simulink model "System_model_discrete"  (R2022a)
settings: Solver=FixedStepDiscrete  StartTime=0.0  StopTime=T_final  FixedStep=T_sample  RelTol=1e-3
values from neighbouring files (symbols this model uses):
  A1 = inv(S1)*IO*U_i.'    [run_model.m]    (also in run_model_for_perform_vs_num_attack.m)
  A2 = OI*U_i.'    [run_model.m]    (also in run_model_for_perform_vs_num_attack.m)
  A_bar_d = [0.99058344787 -0.000125476588979 -1.03572369058e-05 -0.000112840130565 -4.9197018367e-06 -1.67662830632 -0.0228026014464 -0.00188074381714 -0.019999276241 -0.0008715203213 -0.00015214348792 0.987594206485 ... (100 elements, 10x10)]    [A_bar_d.mat]
  b1p = inv(S1)*IO*U_history.'    [run_model.m]    (also in run_model_for_perform_vs_num_attack.m)
  b2p = OI*U_history.'    [run_model.m]    (also in run_model_for_perform_vs_num_attack.m)
  B_bar_d = [0.00129291786986 -6.71376007658e-08 -5.54322132914e-09 -6.10354899312e-08 -2.66151497743e-09 0.269747891814 -1.80552874589e-05 -1.49023321753e-06 -1.61887101691e-05 -7.05777435188e-07 -6.71376007665e-08 0.00108984615129 ... (190 elements, 10x19)]    [B_bar_d.mat]
  BDD_thresh = 0.05*0.6352    (= 0.03176)    [plot_perform_vs_num_attacks.m]    (also in run_model.m)
  C_obsv_d = [0 0 0 0 0 -18.3910466782 17.2834976586 0.26596429707 7.1412513587 0.0956721531682 0.757058744511 -7.14197878204 ... (190 elements, 19x10)]    [C_obsv_d.mat]
  D_obsv_d = [0 0 0 0 0 0 0 0 0 0 0 0 ... (361 elements, 19x19)]    [D_obsv_d.mat]
  e_ini_matrix = reshape(e_ini,n_meas,T1)    [run_model.m]    (also in run_model_for_perform_vs_num_attack.m)
  I = Ic +mc*d^2+2*mw*L^2+2*Im    (= 0.26903125)    [Run_this_file_for_DDWMR_model.m]    (also in run_model.m = [1;2;9;11;12;16;17]; run_model_for_perform_vs_num_attack.m = sort(randperm(n_meas,n_attack)).'; test_different_horizon_size.m = sort(randperm(n_meas,n_attack)).')
  I_attack_ini = repmat(I,1,T1)    [run_model.m]    (also in run_model_for_perform_vs_num_attack.m)
  l = n_meas    (= 19)    [run_model.m]
  load_buses = [zeros(n_gen,1); ones(n_bus-n_gen,1)]    [run_model.m]
  max_iter = 1000    [MHFDIA_Basics.m]    (also in Perform_vs_iter.m = Max_iter(idx); run_model.m = 2000; run_model_for_perform_vs_num_attack.m = 300)
  n = 5    [MHFDIA_Basics.m]    (also in discretize_linear_model.m = size(A,1); run_model.m = 10)
  n_bus = 14    [run_model.m]
  n_gen = 5    [run_model.m]
  n_meas = n_gen + n_bus    (= 19)    [run_model.m]    (also in test_different_horizon_size.m)
  Se1 = S(1:n_states,1:n_states)    [run_model.m]    (also in run_model_for_perform_vs_num_attack.m)
  T = floor(n_x/m)    [MHFDIA_Basics.m]    (also in plot_for_different_horizon_size.m = 20; run_model.m = round(2*n))
  T1 = 20    [plot_perform_vs_num_attacks.m]    (also in run_model.m; test_different_horizon_size.m = T1_array(iter))
  T_start_attack = .2*T_final    [plot_results.m]    (also in run_model.m = 1.6)
  U0 = zeros(m,T)    [run_model.m]
  Ue11 = U(I_attack(1:(T1-1)*n_attack),1:n)    [run_model.m]    (also in run_model_for_perform_vs_num_attack.m)
  Ue12 = U(I_attack((T1-1)*n_attack+1:end),1:n)    [run_model.m]    (also in run_model_for_perform_vs_num_attack.m)
  x0 = zeros(n_states,1)    [run_model.m]
  Y0 = zeros(m,T)    [run_model.m]
undefined symbols (not defined in the file or in its folder): G_T, HT, PhiT, sigbuilder_block, T_start_opt, Theta_T
libraries: simulink x5
settings Model: Creator=oanubi  LastModifiedBy=Abelb
settings SolverCC: AlgebraicLoopSolver=TrustRegion
settings DebuggingCC: UnconnectedInputMsg=warning  UnconnectedOutputMsg=warning  UnconnectedLineMsg=warning  SFMachineParentedDataDiag=warning
settings HardwareCC: TargetBitPerPointer=64  TargetBitPerSizeT=64  TargetBitPerPtrDiffT=64  TargetLongLongMode=on  TargetIntDivRoundTo=Zero  TargetEndianess=LittleEndian  TargetWordSize=64  TargetHWDeviceType=MATLAB Host  ProdEqTarget=off
settings RTWCC: Description=Create Visual C/C++ Solution File for Simulink Coder  TemplateMakefile=RTW.MSVCBuild  DLArmComputeVersion=19.05

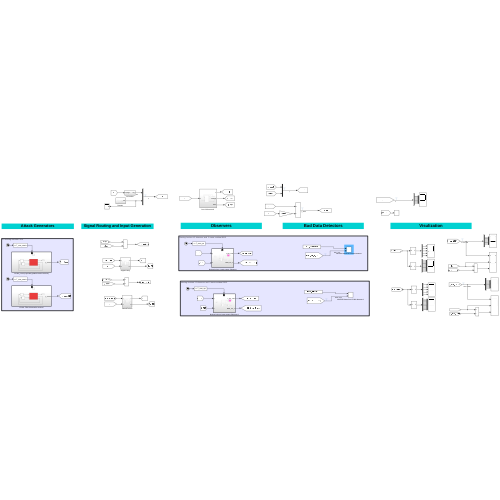
[thumbnail: Simulink's stored preview of the top-level diagram]
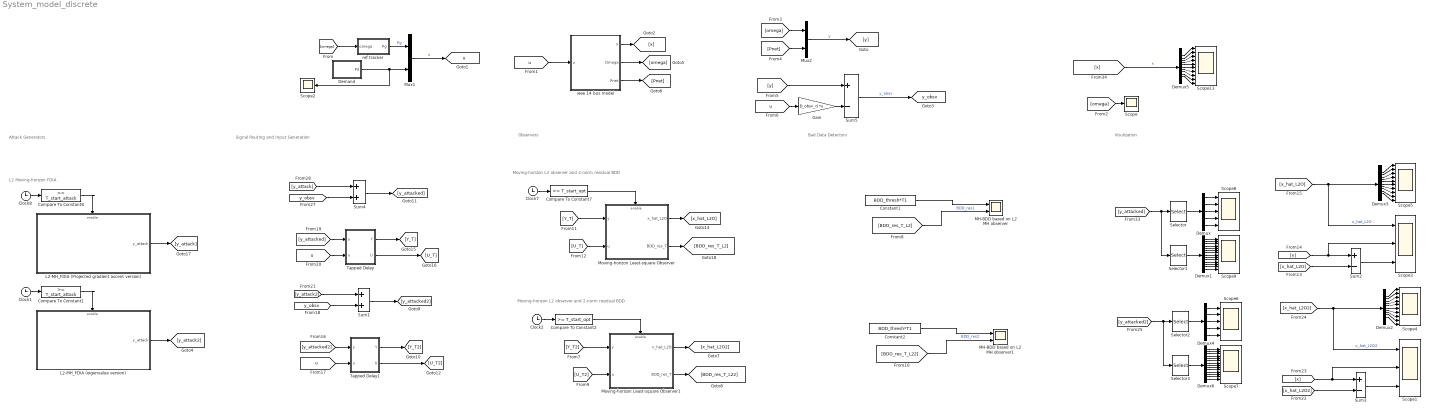
== system System_model_discrete ==
  note: L2 Moving-horizon FDIA
  note: Moving-horizon L2 observer and 2-norm residual BDD
  note: Observers
  note: Signal Routing and Input Generation
  note: Visulization
  note: Attack Generators
  note: Bad Data Detectors
  note: Moving-horizon L2 observer and 2-norm residual BDD
  Clock{1..2,7..8} (4 alike) : Clock
  Compare To Constant1 : simulink/Logic and Bit Operations/Compare To Constant  relop=>=  const=T_start_attack  OutDataTypeStr=boolean
  Compare To Constant2 : simulink/Logic and Bit Operations/Compare To Constant  relop=>=  const=T_start_opt  OutDataTypeStr=boolean
  Compare To Constant7 : simulink/Logic and Bit Operations/Compare To Constant  relop=>=  const=T_start_opt  OutDataTypeStr=boolean
  Compare To Constant8 : simulink/Logic and Bit Operations/Compare To Constant  relop=>=  const=T_start_attack  OutDataTypeStr=boolean
  Constant1 : Constant  Value=BDD_thresh*T1
  Constant2 : Constant  Value=BDD_thresh*T1
  Demand : Subsystem
  Demux : Demux  Outputs=n_gen
  Demux1 : Demux  Outputs=n_bus
  Demux2 : Demux  Outputs=n_states
  Demux3 : Demux  Outputs=n_states
  Demux4 : Demux  Outputs=n_gen
  Demux5 : Demux  Outputs=n_states
  Demux6 : Demux  Outputs=n_bus
  Gain : Gain  Gain=D_obsv_d  Multiplication=Matrix(K*u) (u vector)
  L2-MH_FDIA (Projected gradient ascent version) : Subsystem
  L2-MH_FDIA (eigenvalue version) : Subsystem
  MH-BDD based on L2 MH observer : Scope  NumInputPorts=2
  MH-BDD based on L2 MH observer1 : Scope  NumInputPorts=2
  Moving-horizon Least-square Observer : Subsystem
  Moving-horizon Least-square Observer1 : Subsystem
  Mux1 : Mux  Inputs=2
  Mux2 : Mux  Inputs=2
  Scope : Scope
  Scope1 : Scope  NumInputPorts=3
  Scope13 : Scope  NumInputPorts=10
  Scope2 : Scope
  Scope3 : Scope  NumInputPorts=3
  Scope4 : Scope  NumInputPorts=10
  Scope5 : Scope  NumInputPorts=10
  Scope6 : Scope  NumInputPorts=5
  Scope7 : Scope  NumInputPorts=14
  Scope8 : Scope  NumInputPorts=5
  Scope9 : Scope  NumInputPorts=14
  Selector : Selector  InputPortWidth=n_meas  IndexOptions=Index vector (dialog)  Indices=1:n_gen  OutputSizes=1
  Selector1 : Selector  InputPortWidth=n_meas  IndexOptions=Index vector (dialog)  Indices=n_gen+1:n_meas  OutputSizes=1
  Selector2 : Selector  InputPortWidth=n_meas  IndexOptions=Index vector (dialog)  Indices=1:n_gen  OutputSizes=1
  Selector3 : Selector  InputPortWidth=n_meas  IndexOptions=Index vector (dialog)  Indices=n_gen+1:n_meas  OutputSizes=1
  Sum1 : Sum
  Sum2 : Sum  Inputs=+-
  Sum3 : Sum  Inputs=+-
  Sum4 : Sum
  Sum5 : Sum  Inputs=+-
  Tapped Delay : Subsystem
  Tapped Delay1 : Subsystem
  ieee 14 bus model : Subsystem
  ref tracker : Subsystem
  tag scope: u=global, y_obsv=global
  wires:
  [u] -> ieee 14 bus model/1(u)
  Demand/1(Pd) -> Scope2/1, Mux1/2
  ref tracker/1(Pg) -> Mux1/1  "Pg"
  Mux1/1 -> [u]  "u"
  ieee 14 bus model/2(Omega) -> [omega]
  ieee 14 bus model/1(x) -> [x]
  ieee 14 bus model/3(Pnet) -> [Pnet]
  [omega] -> ref tracker/1(omega)
  [omega] -> Scope/1
  Mux2/1 -> [y]  "y"
  [omega] -> Mux2/1
  [Pnet] -> Mux2/2
  [y] -> Sum5/1
  Gain/1 -> Sum5/2
  [u] -> Gain/1
  Sum5/1 -> [y_obsv]  "y_obsv"
  [y_attacked] -> Tapped Delay/1(y)
  [u] -> Tapped Delay/2(u)
  [y_obsv] -> Sum4/2
  Sum4/1 -> [y_attacked]
  [y_attack] -> Sum4/1
  [y_attacked] -> Selector1/1, Selector/1
  Demux/1 -> Scope8/1
  Demux/2 -> Scope8/2
  Demux/3 -> Scope8/3
  Demux/4 -> Scope8/4
  Demux/5 -> Scope8/5
  Selector/1 -> Demux/1
  Selector1/1 -> Demux1/1
  Demux1/5 -> Scope9/5
  Demux1/4 -> Scope9/4
  Demux1/3 -> Scope9/3
  Demux1/2 -> Scope9/2
  Demux1/1 -> Scope9/1
  Demux1/6 -> Scope9/6
  Demux1/7 -> Scope9/7
  Demux1/8 -> Scope9/8
  Demux1/9 -> Scope9/9
  Demux1/10 -> Scope9/10
  Demux1/11 -> Scope9/11
  Demux1/12 -> Scope9/12
  Demux1/13 -> Scope9/13
  Demux1/14 -> Scope9/14
  [x] -> Demux5/1  "x"
  Demux5/10 -> Scope13/10
  Demux5/6 -> Scope13/6
  Demux5/8 -> Scope13/8
  Demux5/5 -> Scope13/5
  Demux5/3 -> Scope13/3
  Demux5/7 -> Scope13/7
  Demux5/2 -> Scope13/2
  Demux5/1 -> Scope13/1
  Demux5/4 -> Scope13/4
  Demux5/9 -> Scope13/9
  Compare To Constant7/1 -> Moving-horizon Least-square Observer/Enable
  Clock7/1 -> Compare To Constant7/1
  Moving-horizon Least-square Observer/1(x_hat_L2O) -> [x_hat_L2O]
  [x] -> Sum2/1, Scope3/2
  Demux3/3 -> Scope5/3
  Demux3/9 -> Scope5/9
  Demux3/5 -> Scope5/5
  Demux3/7 -> Scope5/7
  Demux3/6 -> Scope5/6
  Demux3/2 -> Scope5/2
  Demux3/1 -> Scope5/1
  Demux3/4 -> Scope5/4
  Demux3/10 -> Scope5/10
  Sum2/1 -> Scope3/3
  Demux3/8 -> Scope5/8
  [x_hat_L2O] -> Demux3/1, Scope3/1  "x_hat_L2O"
  [x_hat_L2O] -> Sum2/2
  Tapped Delay/1(Y) -> [Y_T]
  Tapped Delay/2(U) -> [U_T]
  [Y_T] -> Moving-horizon Least-square Observer/1(y)
  [U_T] -> Moving-horizon Least-square Observer/2(u)
  Moving-horizon Least-square Observer/2(BDD_res_T) -> [BDD_res_T_L2]
  Constant1/1 -> MH-BDD based on L2 MH observer/1
  [BDD_res_T_L2] -> MH-BDD based on L2 MH observer/2  "BDD_res1"
  L2-MH_FDIA (Projected gradient ascent version)/1(y_attack) -> [y_attack]
  Clock8/1 -> Compare To Constant8/1
  Compare To Constant8/1 -> L2-MH_FDIA (Projected gradient ascent version)/Enable
  L2-MH_FDIA (eigenvalue version)/1(y_attack) -> [y_attack2]
  Clock1/1 -> Compare To Constant1/1
  Compare To Constant1/1 -> L2-MH_FDIA (eigenvalue version)/Enable
  [U_T2] -> Moving-horizon Least-square Observer1/2(u)
  Moving-horizon Least-square Observer1/1(x_hat_L2O) -> [x_hat_L2O2]
  Moving-horizon Least-square Observer1/2(BDD_res_T) -> [BDD_res_T_L22]
  Clock2/1 -> Compare To Constant2/1
  [Y_T2] -> Moving-horizon Least-square Observer1/1(y)
  Compare To Constant2/1 -> Moving-horizon Least-square Observer1/Enable
  [BDD_res_T_L22] -> MH-BDD based on L2 MH observer1/2  "BDD_res2"
  Constant2/1 -> MH-BDD based on L2 MH observer1/1
  [y_attack2] -> Sum1/1
  [y_attacked2] -> Tapped Delay1/1(y)
  [u] -> Tapped Delay1/2(u)
  Sum1/1 -> [y_attacked2]
  Tapped Delay1/2(U) -> [U_T2]
  Tapped Delay1/1(Y) -> [Y_T2]
  [y_obsv] -> Sum1/2
  Demux2/10 -> Scope4/10
  [x_hat_L2O2] -> Sum3/2
  [x_hat_L2O2] -> Demux2/1, Scope1/1  "x_hat_L2O2"
  Sum3/1 -> Scope1/3
  [x] -> Sum3/1, Scope1/2
  Demux2/2 -> Scope4/2
  Demux2/7 -> Scope4/7
  Demux2/9 -> Scope4/9
  Demux2/5 -> Scope4/5
  Demux2/8 -> Scope4/8
  Demux2/3 -> Scope4/3
  Demux2/6 -> Scope4/6
  Demux2/1 -> Scope4/1
  Demux2/4 -> Scope4/4
  Demux6/1 -> Scope7/1
  Demux6/13 -> Scope7/13
  Demux4/2 -> Scope6/2
  Demux6/10 -> Scope7/10
  Demux4/4 -> Scope6/4
  Demux6/14 -> Scope7/14
  Demux6/2 -> Scope7/2
  Demux6/12 -> Scope7/12
  Demux6/6 -> Scope7/6
  Demux6/4 -> Scope7/4
  Demux6/11 -> Scope7/11
  Demux6/9 -> Scope7/9
  Demux6/8 -> Scope7/8
  Demux6/5 -> Scope7/5
  Demux4/5 -> Scope6/5
  Selector3/1 -> Demux6/1
  Demux4/1 -> Scope6/1
  Demux4/3 -> Scope6/3
  [y_attacked2] -> Selector3/1, Selector2/1
  Demux6/7 -> Scope7/7
  Demux6/3 -> Scope7/3
  Selector2/1 -> Demux4/1

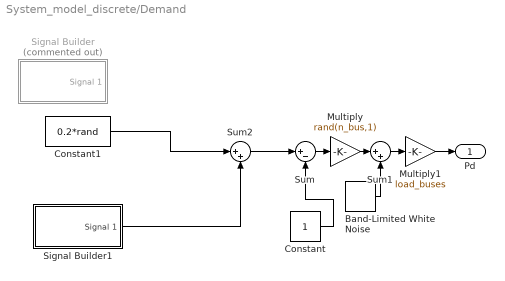
== system System_model_discrete/Demand ==
  Band-Limited White Noise : simulink/Sources/Band-Limited White Noise  Cov=1e-8  Ts=0.1  seed=[23341]
  Constant : Constant
  Constant1 : Constant  Value=0.2*rand
  Multiply : Gain  Gain=rand(n_bus,1)
  Multiply1 : Gain  Gain=load_buses
  Signal Builder : Subsystem  Tag=STV Subsys  Commented=on  LoadFcn=sigbuilder_block('load');  StartFcn=sigbuilder_block('start');  StopFcn=sigbuilder_block('stop');  ClipboardFcn=sigbuilder_block('clipboard');  mask(Sigbuilder block){tuvar=[0:10]}
      mask help: Simulink:masks:SigbuilderBlock_MD
      mask init:
      | if ~strcmp(get_param(bdroot(gcbh),'SimulationStatus'),'stopped') tuvar = sigbuilder_block('maskInit'); end
      settings: CopyFcn=sigbuilder_block('copy');  DeleteFcn=sigbuilder_block('delete');  ModelCloseFcn=sigbuilder_block('modelClose');  PreSaveFcn=sigbuilder_block('preSave');  PauseFcn=sigbuilder_block('pause');  ContinueFcn=sigbuilder_block('continue');  NameChangeFcn=sigbuilder_block('namechange');  OpenFcn=sigbuilder_block('open',[439.2 145.2 550.2 399.9 ]);  CloseFcn=sigbuilder_block('close');
      mask Display: plot(0, 0, 100, 100,[2, 2, 32, 32, 2], [68, 8, 8, 68, 68],[32, 2], [38, 38], [32, 19, 2],[53, 60, 44], [32, 17, 17, 2],[16, 16, 31, 31]);txt = getActiveGroup(gcbh);text(2, 100, txt,'verticalAlignment', 'top');
  Signal Builder1 : Subsystem  Tag=STV Subsys  LoadFcn=sigbuilder_block('load');  StartFcn=sigbuilder_block('start');  StopFcn=sigbuilder_block('stop');  ClipboardFcn=sigbuilder_block('clipboard');  mask(Sigbuilder block){tuvar=[0:10]}
      mask help: Simulink:masks:SigbuilderBlock_MD
      mask init:
      | if ~strcmp(get_param(bdroot(gcbh),'SimulationStatus'),'stopped') tuvar = sigbuilder_block('maskInit'); end
      settings: CopyFcn=sigbuilder_block('copy');  DeleteFcn=sigbuilder_block('delete');  ModelCloseFcn=sigbuilder_block('modelClose');  PreSaveFcn=sigbuilder_block('preSave');  PauseFcn=sigbuilder_block('pause');  ContinueFcn=sigbuilder_block('continue');  NameChangeFcn=sigbuilder_block('namechange');  OpenFcn=sigbuilder_block('open',[439.2 145.2 550.2 399.9 ]);  CloseFcn=sigbuilder_block('close');
      mask Display: plot(0, 0, 100, 100,[2, 2, 32, 32, 2], [68, 8, 8, 68, 68],[32, 2], [38, 38], [32, 19, 2],[53, 60, 44], [32, 17, 17, 2],[16, 16, 31, 31]);txt = getActiveGroup(gcbh);text(2, 100, txt,'verticalAlignment', 'top');
  Sum : Sum  Inputs=|+-
  Sum1 : Sum  Inputs=|++
  Sum2 : Sum  Inputs=|++
  Pd : Outport
  wires:
  Sum/1 -> Multiply/1
  Constant/1 -> Sum/2
  Multiply/1 -> Sum1/1
  Band-Limited White Noise/1 -> Sum1/2
  Sum1/1 -> Multiply1/1
  Multiply1/1 -> Pd/1
  Signal Builder1/1(Signal 1) -> Sum2/2
  Constant1/1 -> Sum2/1
  Sum2/1 -> Sum/1

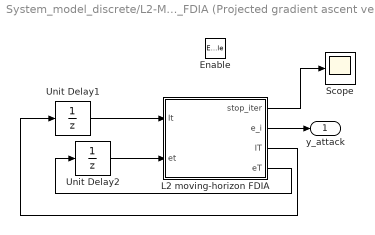
== system System_model_discrete/L2-MH_FDIA (Projected gradient ascent version) ==
  Enable : EnablePort
  L2 moving-horizon FDIA : MATLAB Function  TreatAsAtomicUnit=on
  Scope : Scope
  Unit Delay1 : UnitDelay  InitialCondition=I_attack_ini  SampleTime=-1  HasFrameUpgradeWarning=on
  Unit Delay2 : UnitDelay  InitialCondition=e_ini_matrix  SampleTime=-1  HasFrameUpgradeWarning=on
  y_attack : Outport
  wires:
  L2 moving-horizon FDIA/2(e_i) -> y_attack/1
  Unit Delay1/1 -> L2 moving-horizon FDIA/1(It)
  Unit Delay2/1 -> L2 moving-horizon FDIA/2(et)
  L2 moving-horizon FDIA/3(IT) -> Unit Delay1/1
  L2 moving-horizon FDIA/4(eT) -> Unit Delay2/1
  L2 moving-horizon FDIA/1(stop_iter) -> Scope/1

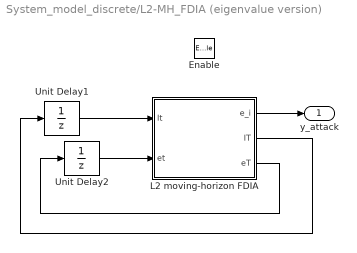
== system System_model_discrete/L2-MH_FDIA (eigenvalue version) ==
  Enable : EnablePort
  L2 moving-horizon FDIA : MATLAB Function  TreatAsAtomicUnit=on
  Unit Delay1 : UnitDelay  InitialCondition=I_attack_ini  SampleTime=-1  HasFrameUpgradeWarning=on
  Unit Delay2 : UnitDelay  InitialCondition=e_ini_matrix  SampleTime=-1  HasFrameUpgradeWarning=on
  y_attack : Outport
  wires:
  L2 moving-horizon FDIA/1(e_i) -> y_attack/1
  Unit Delay1/1 -> L2 moving-horizon FDIA/1(It)
  Unit Delay2/1 -> L2 moving-horizon FDIA/2(et)
  L2 moving-horizon FDIA/2(IT) -> Unit Delay1/1
  L2 moving-horizon FDIA/3(eT) -> Unit Delay2/1

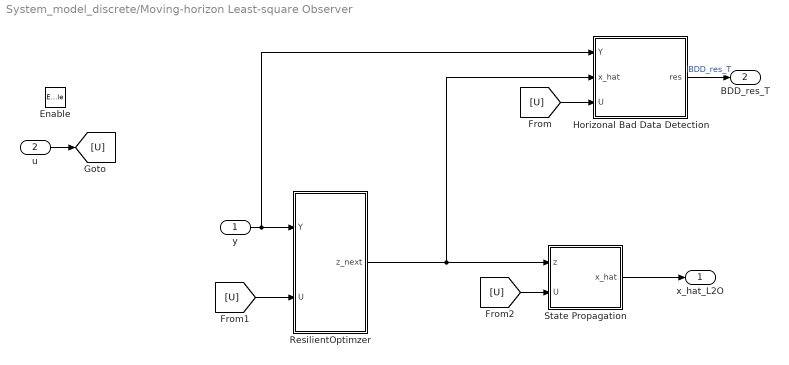
== system System_model_discrete/Moving-horizon Least-square Observer ==
  y : Inport
  u : Inport  Port=2
  Enable : EnablePort
  Horizonal Bad Data Detection : MATLAB Function  TreatAsAtomicUnit=on
  ResilientOptimzer : MATLAB Function  TreatAsAtomicUnit=on
  State Propagation : MATLAB Function  TreatAsAtomicUnit=on
  x_hat_L2O : Outport
  BDD_res_T : Outport  Port=2
  wires:
  y/1 -> Horizonal Bad Data Detection/1(Y), ResilientOptimzer/1(Y)
  State Propagation/1(x_hat) -> x_hat_L2O/1
  ResilientOptimzer/1(z_next) -> Horizonal Bad Data Detection/2(x_hat), State Propagation/1(z)
  u/1 -> [U]
  [U] -> Horizonal Bad Data Detection/3(U)
  [U] -> ResilientOptimzer/2(U)
  [U] -> State Propagation/2(U)
  Horizonal Bad Data Detection/1(res) -> BDD_res_T/1  "BDD_res_T"

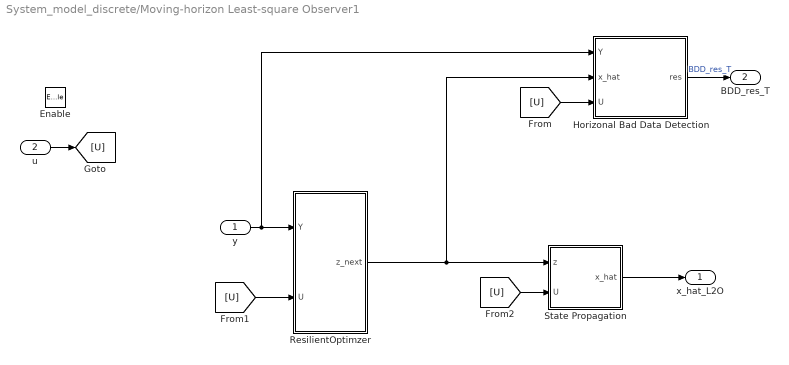
== system System_model_discrete/Moving-horizon Least-square Observer1 ==
  y : Inport
  u : Inport  Port=2
  Enable : EnablePort
  Horizonal Bad Data Detection : MATLAB Function  TreatAsAtomicUnit=on
  ResilientOptimzer : MATLAB Function  TreatAsAtomicUnit=on
  State Propagation : MATLAB Function  TreatAsAtomicUnit=on
  x_hat_L2O : Outport
  BDD_res_T : Outport  Port=2
  wires:
  y/1 -> Horizonal Bad Data Detection/1(Y), ResilientOptimzer/1(Y)
  State Propagation/1(x_hat) -> x_hat_L2O/1
  ResilientOptimzer/1(z_next) -> Horizonal Bad Data Detection/2(x_hat), State Propagation/1(z)
  u/1 -> [U]
  [U] -> Horizonal Bad Data Detection/3(U)
  [U] -> ResilientOptimzer/2(U)
  [U] -> State Propagation/2(U)
  Horizonal Bad Data Detection/1(res) -> BDD_res_T/1  "BDD_res_T"

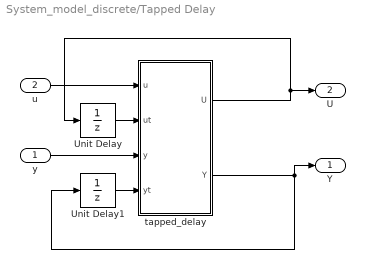
== system System_model_discrete/Tapped Delay ==
  y : Inport
  u : Inport  Port=2
  Unit Delay : UnitDelay  InitialCondition=U0  SampleTime=-1  HasFrameUpgradeWarning=on
  Unit Delay1 : UnitDelay  InitialCondition=Y0  SampleTime=-1  HasFrameUpgradeWarning=on
  tapped_delay : MATLAB Function  TreatAsAtomicUnit=on
  Y : Outport
  U : Outport  Port=2
  wires:
  u/1 -> tapped_delay/1(u)
  y/1 -> tapped_delay/3(y)
  tapped_delay/1(U) -> Unit Delay/1, U/1
  tapped_delay/2(Y) -> Y/1, Unit Delay1/1
  Unit Delay/1 -> tapped_delay/2(ut)
  Unit Delay1/1 -> tapped_delay/4(yt)

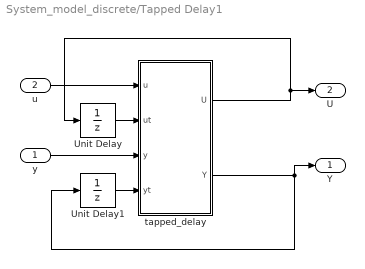
== system System_model_discrete/Tapped Delay1 ==
  y : Inport
  u : Inport  Port=2
  Unit Delay : UnitDelay  InitialCondition=U0  SampleTime=-1  HasFrameUpgradeWarning=on
  Unit Delay1 : UnitDelay  InitialCondition=Y0  SampleTime=-1  HasFrameUpgradeWarning=on
  tapped_delay : MATLAB Function  TreatAsAtomicUnit=on
  Y : Outport
  U : Outport  Port=2
  wires:
  u/1 -> tapped_delay/1(u)
  y/1 -> tapped_delay/3(y)
  tapped_delay/1(U) -> Unit Delay/1, U/1
  tapped_delay/2(Y) -> Y/1, Unit Delay1/1
  Unit Delay/1 -> tapped_delay/2(ut)
  Unit Delay1/1 -> tapped_delay/4(yt)

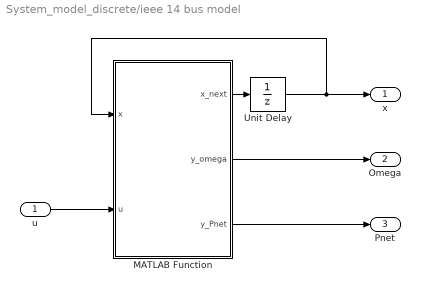
== system System_model_discrete/ieee 14 bus model ==
  u : Inport
  MATLAB Function : MATLAB Function  TreatAsAtomicUnit=on
  Unit Delay : UnitDelay  InitialCondition=x0  SampleTime=-1  HasFrameUpgradeWarning=on
  x : Outport
  Omega : Outport  Port=2
  Pnet : Outport  Port=3
  wires:
  MATLAB Function/1(x_next) -> Unit Delay/1
  u/1 -> MATLAB Function/2(u)
  MATLAB Function/2(y_omega) -> Omega/1
  MATLAB Function/3(y_Pnet) -> Pnet/1
  Unit Delay/1 -> MATLAB Function/1(x), x/1

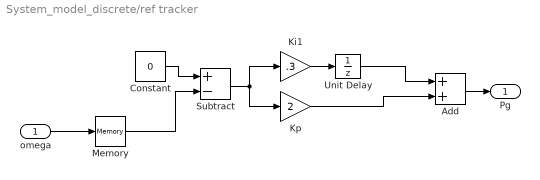
== system System_model_discrete/ref tracker ==
  omega : Inport
  Add : Sum
  Constant : Constant  Value=0
  Ki1 : Gain  Gain=.3
  Kp : Gain  Gain=2
  Memory : Memory  InitialCondition=zeros(n_gen,1)
  Subtract : Sum  Inputs=+-
  Unit Delay : UnitDelay  InitialCondition=zeros(n_gen,1)  SampleTime=-1  HasFrameUpgradeWarning=on
  Pg : Outport
  wires:
  Kp/1 -> Add/2
  Unit Delay/1 -> Add/1
  Add/1 -> Pg/1
  Constant/1 -> Subtract/1
  Subtract/1 -> Ki1/1, Kp/1
  Ki1/1 -> Unit Delay/1
  Memory/1 -> Subtract/2
  omega/1 -> Memory/1

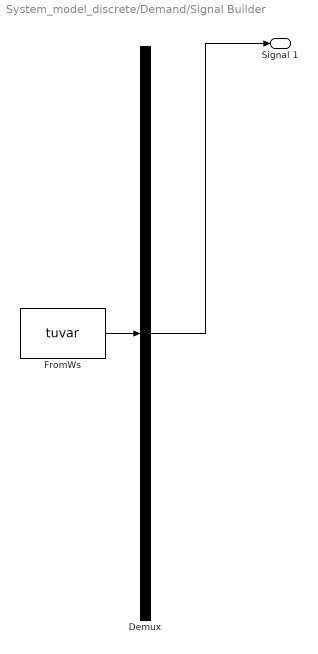
== system System_model_discrete/Demand/Signal Builder ==
  Demux : Demux  Tag=STV Demux  Outputs=1
      settings: DisplayOption=none
  FromWs : FromWorkspace  Tag=STV FromWs  VariableName=tuvar
      SigBuilderData=|
      | common.afterFinalStr = 'Extrapolate'
      | common.sampleTime = 0
      | dataSet.timeRange = [0 10]
      | dataSet.name = 'Group 1'
      | sbobj.Groups.Name = 'Group 1'
      | sbobj.Groups.Signals.Name = 'Signal 1'
      | sbobj.Groups.Signals.XData = [0 0.46 1.5 2.5 4 5 6 7 10]
      | sbobj.Groups.Signals.YData = [1 1.106 1.2 1.2 0.8 0.8 1 1 1]
  Signal 1 : Outport  Tag=STV Outport
  wires:
  Demux/1 -> Signal 1/1
  FromWs/1 -> Demux/1

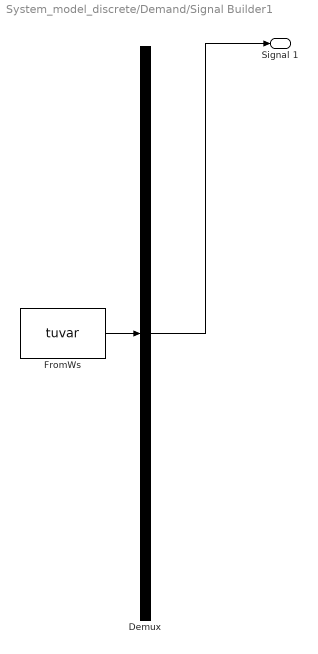
== system System_model_discrete/Demand/Signal Builder1 ==
  Demux : Demux  Tag=STV Demux  Outputs=1
      settings: DisplayOption=none
  FromWs : FromWorkspace  Tag=STV FromWs  VariableName=tuvar
      SigBuilderData=|
      | common.afterFinalStr = 'Extrapolate'
      | common.sampleTime = 0
      | dataSet.timeRange = [0 10]
      | dataSet.name = 'Group 1'
      | sbobj.Groups.Name = 'Group 1'
      | sbobj.Groups.Signals.Name = 'Signal 1'
      | sbobj.Groups.Signals.XData = [0 10]
      | sbobj.Groups.Signals.YData = [0.9 0.9]
  Signal 1 : Outport  Tag=STV Outport
  wires:
  Demux/1 -> Signal 1/1
  FromWs/1 -> Demux/1

== matlab function System_model_discrete/Tapped Delay1/tapped_delay ==
  data: u input; U output; ut input; y input; yt input; Y output
function [U,Y] = fcn(u,ut,y,yt)
%% tapped_delay_array
% shift columns from tapped matrix to the left and appends most recent
% vector to the last column
%%% input
ut(:,1:end-1) = ut(:,2:end);
ut(:,end) = u;
U = ut;
%%% attacked output
yt(:,1:end-1) = yt(:,2:end);
yt(:,end) = y;
Y = yt;

== matlab function System_model_discrete/Tapped Delay/tapped_delay ==
  data: u input; U output; ut input; y input; yt input; Y output
function [U,Y] = fcn(u,ut,y,yt)
%% tapped_delay_array
% shift columns from tapped matrix to the left and appends most recent
% vector to the last column
%%% input
ut(:,1:end-1) = ut(:,2:end);
ut(:,end) = u;
U = ut;
%%% attacked output
yt(:,1:end-1) = yt(:,2:end);
yt(:,end) = y;
Y = yt;

== matlab function System_model_discrete/L2-MH_FDIA (Projected gradient ascent version)/L2 moving-horizon FDIA ==
  data: stop_iter output; A1 parameter; BDD_thresh parameter; It input; et input; T1 parameter; n_meas parameter; A2 parameter; b1p parameter; b2p parameter; e_i output; IT output; eT output; max_iter parameter; I parameter
function [stop_iter,e_i,IT,eT] = fcn(A1,BDD_thresh,It,et, T1, n_meas, A2, b1p, b2p,max_iter,I)
%% generate moving-horizon attack

%% unpacking inputs
et_temp = et(:,2:end);
e_history = et_temp;

It_temp = It(:,2:end);
I_history = It_temp;


%% solve the current attack
I_i = I;  % attack support

[stop_iter,e_i] = L2_MH_FDIA(A1,A2,b1p,b2p,I_history,e_history,I_i,T1,n_meas,T1*BDD_thresh,max_iter);

% eps0 = norm(A2*e_i+b2p*e_history(:));
% eps2 = norm(G2*[et(:);e_i]);
%% store the attack vectors and supports
et(:,1:end-1) = et(:,2:end);
et(:,end) = e_i;
eT = et;
% 
% eps1 = norm(G1*eT(:));


It(:,1:end-1) = It(:,2:end);
It(:,end) = I_i;
IT = It;

== matlab function System_model_discrete/Moving-horizon Least-square Observer/ResilientOptimzer ==
  data: z_next output; Y input; U input; PhiT parameter; l parameter; T parameter; HT parameter
function z_next  = fcn(Y,U, PhiT,l,T,HT)
u_local = zeros(l,T-1);
u_local(:,:) = U(:,1:end-1);
% vectorized
u = u_local(:);
y = Y(:);

%% estimation
z_next = pinv(PhiT,0.01)*(y-HT*u);

== matlab function System_model_discrete/Moving-horizon Least-square Observer/State Propagation ==
  data: z input; U input; x_hat output; Theta_T parameter; n parameter; G_T parameter; T parameter; l parameter
function x_hat = fcn(z,U,Theta_T, n,G_T, T, l)
% x_hat = fcn(z,U,PhiT, HT,n_states)
% Propagates the estimated intial state to the current time
u_local = zeros(l,T-1);
u_local(:,:) = U(:,1:end-1);


% State propagation
x_hat = Theta_T*z(1:n) + G_T*u_local(:);

== matlab function System_model_discrete/Moving-horizon Least-square Observer/Horizonal Bad Data Detection ==
  data: Y input; x_hat input; res output; PhiT parameter; HT parameter; l parameter; T parameter; U input
function res = fcn(Y,x_hat,PhiT,HT, l, T, U)
u_local = zeros(l,T-1);
u_local(:,:) = U(:,1:end-1);
% vectorized
u = u_local(:);
y = Y(:);

res = norm(y-PhiT*x_hat-HT*u,2);

== matlab function System_model_discrete/L2-MH_FDIA (eigenvalue version)/L2 moving-horizon FDIA ==
  data: BDD_thresh parameter; It input; et input; T1 parameter; n_meas parameter; Ue11 parameter; Ue12 parameter; Se1 parameter; e_i output; IT output; eT output; I parameter
function [e_i,IT,eT] = fcn(BDD_thresh,It,et, T1, n_meas, Ue11,Ue12,Se1,I)
%% generate moving-horizon attack

%% unpacking inputs
et_temp = et(:,2:end);
e_history = et_temp;

It_temp = It(:,2:end);
I_history = It_temp;


%% solve the current attack
I_i = I;  % attack support

e_i = L2_MH_FDIA_eigVersion(e_history,I_history, I_i, T1,n_meas,T1*BDD_thresh, Ue11,Ue12,Se1);

% eps0 = norm(A2*e_i+b2p*e_history(:));
% eps2 = norm(G2*[et(:);e_i]);
%% store the attack vectors and supports
et(:,1:end-1) = et(:,2:end);
et(:,end) = e_i;
eT = et;

% eps1 = norm(G1*eT(:));


It(:,1:end-1) = It(:,2:end);
It(:,end) = I_i;
IT = It;

== matlab function System_model_discrete/ieee 14 bus model/MATLAB Function ==
  data: x input; x_next output; u input; y_omega output; A_bar_d parameter; C_obsv_d parameter; B_bar_d parameter; D_obsv_d parameter; n_gen parameter; n_bus parameter; y_Pnet output
function [x_next,y_omega,y_Pnet] = fcn(x,u,A_bar_d,C_obsv_d,B_bar_d,D_obsv_d,n_gen, n_bus)
% Discrete state-space model for system

x_next = A_bar_d*x + B_bar_d*u;

y = C_obsv_d*x + D_obsv_d*u;

y_omega = y(1:n_gen);
y_Pnet = y(n_gen+1:n_bus+n_gen);

== matlab function System_model_discrete/Moving-horizon Least-square Observer1/Horizonal Bad Data Detection ==
  data: Y input; x_hat input; res output; PhiT parameter; HT parameter; l parameter; T parameter; U input
function res = fcn(Y,x_hat,PhiT,HT, l, T, U)
u_local = zeros(l,T-1);
u_local(:,:) = U(:,1:end-1);
% vectorized
u = u_local(:);
y = Y(:);

res = norm(y-PhiT*x_hat-HT*u,2);

== matlab function System_model_discrete/Moving-horizon Least-square Observer1/ResilientOptimzer ==
  data: z_next output; Y input; U input; PhiT parameter; l parameter; T parameter; HT parameter
function z_next  = fcn(Y,U, PhiT,l,T,HT)
u_local = zeros(l,T-1);
u_local(:,:) = U(:,1:end-1);
% vectorized
u = u_local(:);
y = Y(:);

%% estimation
z_next = pinv(PhiT,0.01)*(y-HT*u);

== matlab function System_model_discrete/Moving-horizon Least-square Observer1/State Propagation ==
  data: z input; U input; x_hat output; Theta_T parameter; n parameter; G_T parameter; T parameter; l parameter
function x_hat = fcn(z,U,Theta_T, n,G_T, T, l)
% x_hat = fcn(z,U,PhiT, HT,n_states)
% Propagates the estimated intial state to the current time
u_local = zeros(l,T-1);
u_local(:,:) = U(:,1:end-1);


% State propagation
x_hat = Theta_T*z(1:n) + G_T*u_local(:);
